simulink model "EX2"  (R2023a)
settings: Solver=FixedStepDiscrete  StartTime=0.0  StopTime=100.0  FixedStep=1/1000  RelTol=1e-3  EnableMultiTasking=on
libraries: commanapbnd3 x2, visionstatistics x1, commchan3 x1, dspfdesign x1
settings Model: Creator=Roy  LastModifiedBy=Roy

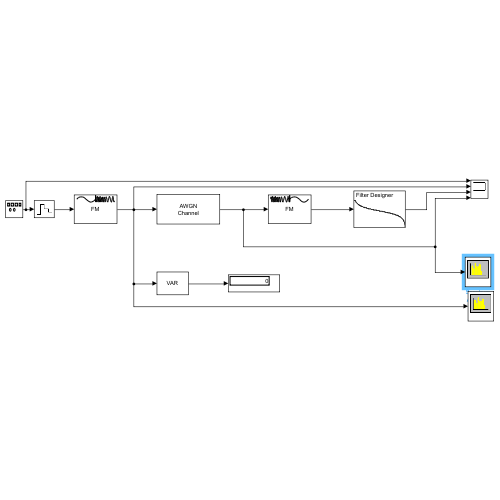
[thumbnail: Simulink's stored preview of the top-level diagram]
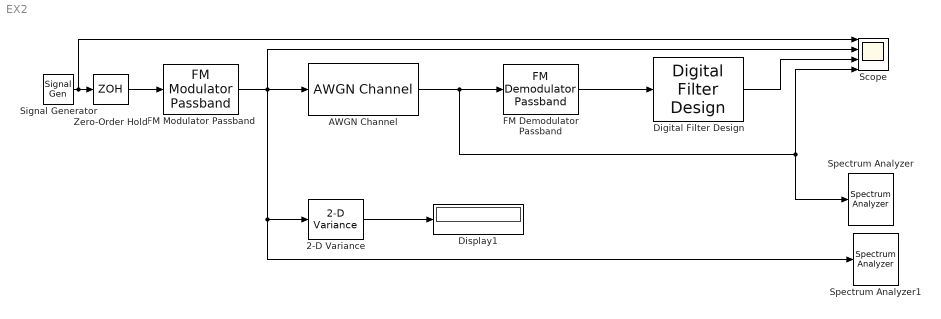
== system EX2 ==
  2-D Variance : visionstatistics/2-D Variance  run=off  reset_popup=None  directionMode=Entire input  dimension=1  treatSBRowAsCol=on  roiEnable=off  roiType=Rectangles  roiPortion=Entire ROI  roiOutput=Individual statistics for each ROI  roiFlag=off  roundingMode=Floor  overflowMode=off  prodOutputMode=Binary point scaling  prodOutputWordLength=32  prodOutputFracLength=0  prodOutputSlope=2^0  memorySlope=2^-30  accumSlope=2^-32  outputSlope=2^-32
  AWGN Channel : commchan3/AWGN Channel  LegacyMode=off  NoiseMethod="Signal to noise ratio  (SNR)"  noiseMode="Signal to noise ratio  (SNR)"  EbNo=10  EsNo=10  SNR=10  BitsPerSymbol=1  SignalPower=0.5  SamplesPerSymbol=1  SymbolPeriod=1  VarianceSource=Parameter  Variance=1  RandomStream=mt19937ar with seed  Seed=67  SimulateUsing=Code generation
  Digital Filter Design : dspfdesign/Digital Filter Design  mwdsp_browser_bugfix_var=off
  Display1 : Display
  FM Demodulator Passband : commanapbnd3/FM Demodulator Passband  Fc=100  Ph=0  Kc=10  Ho=100
  FM Modulator Passband : commanapbnd3/FM Modulator Passband  Fc=100  Ph=0  Kc=10
  Scope : Scope  NumInputPorts=4
  Signal Generator : SignalGenerator  Amplitude=0.5  Frequency=5
  Spectrum Analyzer : SpectrumAnalyzer  WindowPosition=[85.000000,236.000000,800.000000,500.000000,]  ScopeFrameLocation=window  SampleRateSource=Property  SampleRate=44.1e3  PlotAsTwoSidedSpectrum=off  FrequencyScale=Log  FrequencySpan=Start and stop frequencies  StartFrequency=20  StopFrequency=20e3  YLimits=[-22.82571037,29.87460886]  ColorLimits=[-20 80]  DefaultConfigurationName=spbscopes.SpectrumAnalyzerBlockCfg  IsFrequencyInputMode=0  FrequencyVectorPort=0  FrequencyVectorFromPort=0  FrequencyInputRBWPort=0  FrequencyInputRBWFromPort=0
  Spectrum Analyzer1 : SpectrumAnalyzer  WindowPosition=[880.000000,262.000000,800.000000,500.000000,]  ScopeFrameLocation=window  SampleRateSource=Property  SampleRate=44.1e3  PlotAsTwoSidedSpectrum=off  FrequencyScale=Log  FrequencySpan=Start and stop frequencies  StartFrequency=20  StopFrequency=20e3  YLimits=[-81.74415237,36.44007901]  ColorLimits=[-20 80]  DefaultConfigurationName=spbscopes.SpectrumAnalyzerBlockCfg  IsFrequencyInputMode=0  FrequencyVectorPort=0  FrequencyVectorFromPort=0  FrequencyInputRBWPort=0  FrequencyInputRBWFromPort=0
  Zero-Order Hold : ZeroOrderHold  SampleTime=1/1000
  wires:
  Signal Generator/1 -> Scope/1, Zero-Order Hold/1
  Zero-Order Hold/1 -> FM Modulator Passband/1
  FM Modulator Passband/1 -> AWGN Channel/1, Scope/2, Spectrum Analyzer1/1, 2-D Variance/1
  FM Demodulator Passband/1 -> Digital Filter Design/1
  Digital Filter Design/1 -> Scope/3
  AWGN Channel/1 -> Scope/4, Spectrum Analyzer/1, FM Demodulator Passband/1
  2-D Variance/1 -> Display1/1
